simulink model "Trab1_desafio1"  (R2018a)
settings: Solver=VariableStepAuto  StartTime=0.0  StopTime=10.0  FixedStep=0.1  RelTol=1e-4
values from neighbouring files (symbols this model uses):
  A = [0 1 0 0; -K/M 0 K/M 0; 0 0 0 1; K/M 0 -K/M 0]    [Trab1_desafio_1.m]
  B = [0 0; 1/M 0; 0 0; 0 1/M]    [Trab1_desafio_1.m]
  C = [1 0 0 0; 0 0 1 0]    [Trab1_desafio_1.m]
  x0 = [x10; 0; x20; 0]    [Trab1_desafio_1.m]
settings Model: Creator=eric-  LastModifiedBy=eric-

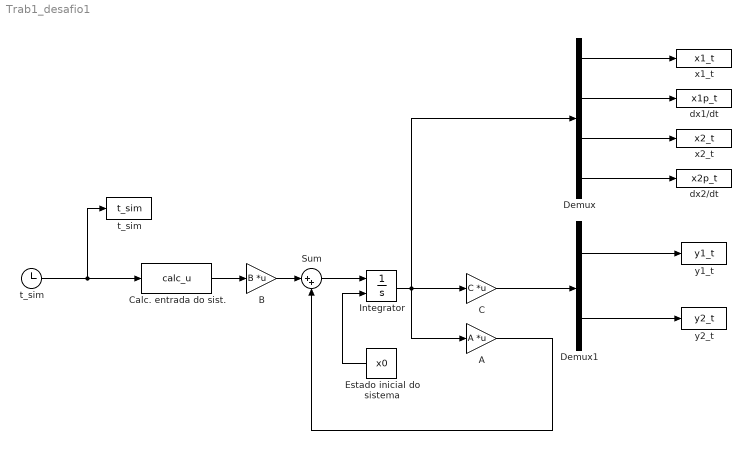
== system Trab1_desafio1 ==
  A : Gain  Gain=A  Multiplication=Matrix(K*u)
  B : Gain  Gain=B  Multiplication=Matrix(K*u)
  C : Gain  Gain=C  Multiplication=Matrix(K*u)
  Calc. entrada do sist. : MATLABFcn  MATLABFcn=calc_u  OutputDimensions=[2 1]  Output1D=off
  Demux : Demux
  Demux1 : Demux  Outputs=2
  Estado inicial do sistema : Constant  Value=x0
  Integrator : Integrator  InitialConditionSource=external  InitialCondition=x0
  Sum : Sum  Inputs=|++
  dx1/dt : ToWorkspace  VariableName=x1p_t  SampleTime=-1
      settings: Save2DSignal=2-D array (concatenate along first dimension)
  dx2/dt : ToWorkspace  VariableName=x2p_t  SampleTime=-1
      settings: Save2DSignal=2-D array (concatenate along first dimension)
  t_sim : ToWorkspace  VariableName=t_sim  SampleTime=-1
      settings: Save2DSignal=2-D array (concatenate along first dimension)
  "t_sim " : Clock
  x1_t : ToWorkspace  VariableName=x1_t  SampleTime=-1
      settings: Save2DSignal=2-D array (concatenate along first dimension)
  x2_t : ToWorkspace  VariableName=x2_t  SampleTime=-1
      settings: Save2DSignal=2-D array (concatenate along first dimension)
  y1_t : ToWorkspace  VariableName=y1_t  SampleTime=-1
      settings: Save2DSignal=2-D array (concatenate along first dimension)
  y2_t : ToWorkspace  VariableName=y2_t  SampleTime=-1
      settings: Save2DSignal=2-D array (concatenate along first dimension)
  wires:
  Sum/1 -> Integrator/1
  A/1 -> Sum/2
  B/1 -> Sum/1
  Integrator/1 -> A/1, C/1, Demux/1
  "t_sim "/1 -> Calc. entrada do sist./1, t_sim/1
  Calc. entrada do sist./1 -> B/1
  Demux/1 -> x1_t/1
  Demux/2 -> dx1/dt/1
  Demux/3 -> x2_t/1
  Demux/4 -> dx2/dt/1
  C/1 -> Demux1/1
  Demux1/1 -> y1_t/1
  Demux1/2 -> y2_t/1
  Estado inicial do sistema/1 -> Integrator/2
